simulink model "laba5_QPSK2"  (R2022a)
settings: Solver=ode45  StartTime=0.0  StopTime=0.128  RelTol=1e-3  EnableMultiTasking=on
libraries: commrandsrc2 x2, commseqgen3 x1
settings Model: Creator=Lenovo  LastModifiedBy=anton
settings SolverCC: AlgebraicLoopSolver=TrustRegion
settings DataIOCC: LimitDataPoints=on  SaveFormat=Array  SignalLoggingSaveFormat=ModelDataLogs  ReturnWorkspaceOutputs=off
settings OptimizationCC: ExpressionDepthLimit=2147483647  LifeSpan=inf
settings DebuggingCC: UnderspecifiedInitializationDetection=Classic  MergeDetectMultiDrivingBlocksExec=none  SolverPrmCheckMsg=warning  FcnCallInpInsideContextMsg=warning  UnconnectedInputMsg=warning  UnconnectedOutputMsg=warning  UnconnectedLineMsg=warning  StateNameClashWarn=warning  SFUnexpectedBacktrackingDiag=warning  SFNoUnconditionalDefaultTransitionDiag=warning  SFExecutionAtInitializationDiag=none  SFMachineParentedDataDiag=warning  ArithmeticOperatorsInVariantConditions=warning
settings HardwareCC: ProdBitPerPointer=32  ProdBitPerSizeT=32  ProdBitPerPtrDiffT=32  ProdLargestAtomicFloat=None  ProdIntDivRoundTo=Undefined  ProdEndianess=Unspecified  ProdWordSize=32  ProdHWDeviceType=32-bit Generic
settings ModelReferenceCC: PropagateSignalLabelsOutOfModel=off
settings SFSimCC: SimUseLocalCustomCode=off  CustomCodeUndefinedFunction=UseInterfaceOnly
settings RTWCC: RTWUseLocalCustomCode=off
settings CodeAppCC: StateflowObjectComments=on
settings GRTTargetCC: TargetLangStandard=C89/C90 (ANSI)  CombineOutputUpdateFcns=off  GRTInterface=on
settings ConfigComp: CovMetricSettings=dw  CovSaveCumulativeToWorkspaceVar=on  CovSaveSingleToWorkspaceVar=on  CovExternalEMLEnable=off

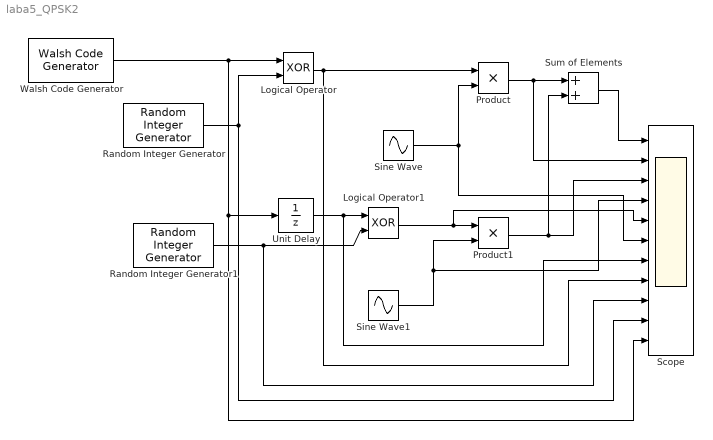
== system laba5_QPSK2 ==
  Logical Operator : Logic  Operator=XOR  AllPortsSameDT=off  OutDataTypeStr=boolean
  Logical Operator1 : Logic  Operator=XOR  AllPortsSameDT=off  OutDataTypeStr=boolean
  Product : Product  RndMeth=Zero
  Product1 : Product  RndMeth=Zero
  Random Integer Generator : commrandsrc2/Random Integer Generator  mul=2  seed=01090  Ts=1/1.2288/10^6  frameBased=off  sampPerFrame=1  orient=off  outDataType=double
      settings: SourceProductBaseCode=CM
  Random Integer Generator1 : commrandsrc2/Random Integer Generator  mul=2  seed=133  Ts=1/1.2288/10^6  frameBased=off  sampPerFrame=1  orient=off  outDataType=double
      settings: SourceProductBaseCode=CM
  Scope : Scope  NumInputPorts=11
  Sine Wave : Sin  SampleTime=0
  Sine Wave1 : Sin  SampleTime=0
  Sum of Elements : Sum
  Unit Delay : UnitDelay  SampleTime=-1
  Walsh Code Generator : commseqgen3/Walsh Code Generator  Length=128  Index=90  SampleTime=1/1.2288/10^6  SamplesPerFrame=1  OutputDataType=double  SimulateUsing=Code generation
      settings: SourceProductBaseCode=CM
  wires:
  Unit Delay/1 -> Logical Operator1/1, Scope/7
  Walsh Code Generator/1 -> Logical Operator/1, Unit Delay/1, Scope/11
  Logical Operator/1 -> Product/1, Scope/8
  Product/1 -> Sum of Elements/1, Scope/2
  Logical Operator1/1 -> Product1/1, Scope/5
  Sine Wave1/1 -> Product1/2, Scope/4
  Sum of Elements/1 -> Scope/1
  Product1/1 -> Scope/3, Sum of Elements/2
  Sine Wave/1 -> Scope/6, Product/2
  Random Integer Generator/1 -> Logical Operator/2, Scope/10
  Random Integer Generator1/1 -> Logical Operator1/2, Scope/9
